simulink model "Pendulum_CAD_Control_R2020a"  (R2020a)
settings: Solver=VariableStepAuto  StartTime=0.0  StopTime=10.0  RelTol=1e-3
values from neighbouring files (symbols this model uses):
  g = 9.81    [Base Variables.mat]
  gain_motor = 5.67    [Base Variables.mat]
  jp = 0.000110755392    [Base Variables.mat]
  lp = 0.1832    [Base Variables.mat]
  M = 0.0203    [Base Variables.mat]
  Mp = 0.0033    [Base Variables.mat]
  R = 0.109    [Base Variables.mat]
undefined symbols (not defined in the file or in its folder): X, Y, Z
libraries: sm_lib x45, nesl_utility x6, fl_lib x4
(part 2 of 2)

== system Pendulum_CAD_Control_R2020a/Plant/h_encoderaxles_1_RIGID/glidewheel_encoder_2_RIGID ==
  Solid : sm_lib/Body Elements/File Solid  ExtGeomFileName=glidewheel_encoder_Default_sldprt.STL  UnitType=Custom  ExtGeomFileUnits=mm  StepReaderType=HEX  ExportConvexHullGeometry=off  InertiaType=Custom  Mass=0.012717581311371812  MassUnits=kg  CenterOfMass=[20 23.311862389290109 3.5000000000000004]  CenterOfMassUnits=mm  MomentsOfInertia=[2.4036537381786549 1.6085577350900775 3.9083512258925288]  MomentsOfInertiaUnits=kg*mm^2  ProductsOfInertia=[0 0 0]  ProductsOfInertiaUnits=kg*mm^2  BasedOnType=Density  Density=1000  DensityUnits=kg/(m^3)  DoExposeReferenceFrame=on  SerializedFrames=<Frames/>  GraphicType=FromGeometry  MarkerShape=Sphere  MarkerSize=10  MarkerSizeUnits=m  GraphicVisPropType=SimpleVisualProperties  GraphicDiffuseColor=[0.4 0.4 0.4]  GraphicSpecularColor=[0.5 0.5 0.5 1.0]  GraphicAmbientColor=[0.15 0.15 0.15 1.0]  GraphicEmissiveColor=[0.0 0.0 0.0 1.0]  GraphicShininess=75  GraphicOpacity=1
  F : PMIOPort  Side=Left
  connections:
  Solid/RConn1 -- F/RConn1

== system Pendulum_CAD_Control_R2020a/Plant/h_encoderaxles_1_RIGID/h_triangle_1_RIGID ==
  Solid : sm_lib/Body Elements/File Solid  ExtGeomFileName=h_triangle_Default_sldprt.STL  UnitType=Custom  ExtGeomFileUnits=mm  StepReaderType=HEX  ExportConvexHullGeometry=off  InertiaType=Custom  Mass=0.0010321252629775849  MassUnits=kg  CenterOfMass=[0 0 -7.5566061536848483]  CenterOfMassUnits=mm  MomentsOfInertia=[0.036987929193085974 0.14119048806599191 0.1060088988565826]  MomentsOfInertiaUnits=kg*mm^2  ProductsOfInertia=[0 0 0]  ProductsOfInertiaUnits=kg*mm^2  BasedOnType=Density  Density=1000  DensityUnits=kg/(m^3)  DoExposeReferenceFrame=on  SerializedFrames=<Frames/>  GraphicType=FromGeometry  MarkerShape=Sphere  MarkerSize=10  MarkerSizeUnits=m  GraphicVisPropType=SimpleVisualProperties  GraphicDiffuseColor=[0.2 0.2 0.2]  GraphicSpecularColor=[0.5 0.5 0.5 1.0]  GraphicAmbientColor=[0.15 0.15 0.15 1.0]  GraphicEmissiveColor=[0.0 0.0 0.0 1.0]  GraphicShininess=75  GraphicOpacity=1
  F : PMIOPort  Side=Left
  connections:
  Solid/RConn1 -- F/RConn1

== system Pendulum_CAD_Control_R2020a/Plant/h_encoderaxles_1_RIGID/x86_axle_4_RIGID ==
  Solid : sm_lib/Body Elements/File Solid  ExtGeomFileName=86_axle_Default_sldprt.STL  UnitType=Custom  ExtGeomFileUnits=mm  StepReaderType=HEX  ExportConvexHullGeometry=off  InertiaType=Custom  Mass=0.0011644908507951884  MassUnits=kg  CenterOfMass=[0 0 0]  CenterOfMassUnits=mm  MomentsOfInertia=[0.0027714374516001608 0.7160611630059921 0.7160611630059921]  MomentsOfInertiaUnits=kg*mm^2  ProductsOfInertia=[0 0 0]  ProductsOfInertiaUnits=kg*mm^2  BasedOnType=Density  Density=1000  DensityUnits=kg/(m^3)  DoExposeReferenceFrame=on  SerializedFrames=<Frames/>  GraphicType=FromGeometry  MarkerShape=Sphere  MarkerSize=10  MarkerSizeUnits=m  GraphicVisPropType=SimpleVisualProperties  GraphicDiffuseColor=[0.4 0.4 0.4]  GraphicSpecularColor=[0.5 0.5 0.5 1.0]  GraphicAmbientColor=[0.15 0.15 0.15 1.0]  GraphicEmissiveColor=[0.0 0.0 0.0 1.0]  GraphicShininess=75  GraphicOpacity=1
  F : PMIOPort  Side=Left
  connections:
  Solid/RConn1 -- F/RConn1

== system Pendulum_CAD_Control_R2020a/Plant/h_encoderaxles_1_RIGID/x86_axle_5_RIGID ==
  Solid : sm_lib/Body Elements/File Solid  ExtGeomFileName=86_axle_Default_sldprt.STL  UnitType=Custom  ExtGeomFileUnits=mm  StepReaderType=HEX  ExportConvexHullGeometry=off  InertiaType=Custom  Mass=0.0011644908507951884  MassUnits=kg  CenterOfMass=[0 0 0]  CenterOfMassUnits=mm  MomentsOfInertia=[0.0027714374516001608 0.7160611630059921 0.7160611630059921]  MomentsOfInertiaUnits=kg*mm^2  ProductsOfInertia=[0 0 0]  ProductsOfInertiaUnits=kg*mm^2  BasedOnType=Density  Density=1000  DensityUnits=kg/(m^3)  DoExposeReferenceFrame=on  SerializedFrames=<Frames/>  GraphicType=FromGeometry  MarkerShape=Sphere  MarkerSize=10  MarkerSizeUnits=m  GraphicVisPropType=SimpleVisualProperties  GraphicDiffuseColor=[0.4 0.4 0.4]  GraphicSpecularColor=[0.5 0.5 0.5 1.0]  GraphicAmbientColor=[0.15 0.15 0.15 1.0]  GraphicEmissiveColor=[0.0 0.0 0.0 1.0]  GraphicShininess=75  GraphicOpacity=1
  F : PMIOPort  Side=Left
  connections:
  Solid/RConn1 -- F/RConn1

== system Pendulum_CAD_Control_R2020a/Plant/h_encoderaxles_1_RIGID/x86_axle_6_RIGID ==
  Solid : sm_lib/Body Elements/File Solid  ExtGeomFileName=86_axle_Default_sldprt.STL  UnitType=Custom  ExtGeomFileUnits=mm  StepReaderType=HEX  ExportConvexHullGeometry=off  InertiaType=Custom  Mass=0.0011644908507951884  MassUnits=kg  CenterOfMass=[0 0 0]  CenterOfMassUnits=mm  MomentsOfInertia=[0.0027714374516001608 0.7160611630059921 0.7160611630059921]  MomentsOfInertiaUnits=kg*mm^2  ProductsOfInertia=[0 0 0]  ProductsOfInertiaUnits=kg*mm^2  BasedOnType=Density  Density=1000  DensityUnits=kg/(m^3)  DoExposeReferenceFrame=on  SerializedFrames=<Frames/>  GraphicType=FromGeometry  MarkerShape=Sphere  MarkerSize=10  MarkerSizeUnits=m  GraphicVisPropType=SimpleVisualProperties  GraphicDiffuseColor=[0.4 0.4 0.4]  GraphicSpecularColor=[0.5 0.5 0.5 1.0]  GraphicAmbientColor=[0.15 0.15 0.15 1.0]  GraphicEmissiveColor=[0.0 0.0 0.0 1.0]  GraphicShininess=75  GraphicOpacity=1
  F : PMIOPort  Side=Left
  connections:
  Solid/RConn1 -- F/RConn1

== matlab function Pendulum_CAD_Control_R2020a/Balance Control/MATLAB Function1 ==
  data: alpha input; alphadot input; y output; beta input; betadot input
function y = balance_control(alpha, alphadot, beta, betadot)
k = [1.4142  -24.7252    1.2178   -2.3548]
y = -k*[alpha;beta;alphadot;betadot]

== matlab function Pendulum_CAD_Control_R2020a/Swing Up/MATLAB Function ==
  data: alphadot input; beta input; torque output; betadot input
function torque = swingup_control(alphadot, beta,betadot)
% M = 20.3e-3; % 0.203
% R = 109e-3;
% mp = 3.3e-3;
% lp = 183.2e-3;
% g = 9.81;
% T = 2*pi*sqrt(lp/g);
% f = 1/T;
% gain_motor = 5.67;
% alpha_up = beta;%-pi
% 
% jp = 1/4*mp*g*lp/(pi^2*f^2);
% T = 1/2*jp*betadot^2;
% U = mp*g*lp*(1-cos(alpha_up));
% E = T+U;
% %u1 = gain_motor*sign(E*betadot*cos(alpha_up))
% u1 = gain_motor*(1/(1+exp(-E*betadot*cos(alpha_up))))
% betadot
% torque_max = 0.1e3;
% torque = M*u1*R;
% % torque = min(torque_max,max(torque,-torque_max));
torque = sign(betadot*cos(beta))*(cos(beta)-1)*0.36
end
